simulink model "mrefrobotarm_modified_previous_y_previous_u_previous_ref_pert_2"  (R2018b)
settings: Solver=FixedStepAuto  StartTime=0.0  StopTime=60  RelTol=1e-3  AbsTol=1e-6
undefined symbols (not defined in the file or in its folder): cc, options
libraries: neural x858, simulink x1
(part 12 of 32)

== system mrefrobotarm_modified_previous_y_previous_u_previous_ref_pert_2/m=0 sd=0.001/Layer 3/Delays 1 ==
  "p{3}" : Inport  PortDimensions=30
      mask Display: e = 0.06;c1 = [120 230 180]/255;c2 = ([120 230 180]+0)/(256+128);c3 = ([120 230 180]+128)/(256+128);patch([0 1 1 0],[0 0 1 1],c1);patch([0 1 1 1-e 1-e 0+e],[0 0 1 1-e 0+e 0+e],c2);patch([0 0 1 1-e 0+e 0+e],[0 1 1 1-e 1-e 0+e],c3);plot([0 1 1 0 0],[0 0 1 1 0]);
  mux : Mux  Inputs=1
      mask Display: e = 0.06;c1 = [120 150 230]/255;c2 = ([120 150 230]+0)/383;c3 = ([120 150 230]+128)/383;patch([0 1 1 0],[0 0 1 1],c1);patch([0 1 1 1-e 1-e 0+e],[0 0 1 1-e 0+e 0+e],c2);patch([0 0 1 1-e 0+e 0+e],[0 1 1 1-e 1-e 0+e],c3);plot([0 1 1 0 0],[0 0 1 1 0]);disp('Mux')
  "pd{3,2}" : Outport
      mask Display: e = 0.06;c1 = [120 230 180]/255;c2 = ([120 230 180]+0)/(256+128);c3 = ([120 230 180]+128)/(256+128);patch([0 1 1 0],[0 0 1 1],c1);patch([0 1 1 1-e 1-e 0+e],[0 0 1 1-e 0+e 0+e],c2);patch([0 0 1 1-e 0+e 0+e],[0 1 1 1-e 1-e 0+e],c3);plot([0 1 1 0 0],[0 0 1 1 0]);
  wires:
  "p{3}"/1 -> mux/1
  mux/1 -> "pd{3,2}"/1

== system mrefrobotarm_modified_previous_y_previous_u_previous_ref_pert_2/m=0 sd=0.001/Layer 3/LW{3,2} ==
  "ad{3,2}" : Inport  PortDimensions=30
      mask Display: e = 0.06;c1 = [120 230 180]/255;c2 = ([120 230 180]+0)/(256+128);c3 = ([120 230 180]+128)/(256+128);patch([0 1 1 0],[0 0 1 1],c1);patch([0 1 1 1-e 1-e 0+e],[0 0 1 1-e 0+e 0+e],c2);patch([0 0 1 1-e 0+e 0+e],[0 1 1 1-e 1-e 0+e],c3);plot([0 1 1 0 0],[0 0 1 1 0]);
  "IW{3,2}(1,:)'" : Constant  Value=[-0.1402055465054231897514824822792434133589267730712890625;-0.010591721623553325415389991803749580867588520050048828125;0.66868572840284390412790571645018644630908966064453125;0.06398114714037583805605891029699705541133880615234375;-0.86465249332831961570633438896038569509983062744140625;0.048965740146590712444929494040479767136275768280029296875;0.047539519471818426910036947674598195590078830718994140625;-0.000811648651889989897374733107682232002844102680683135986328125;-0.07220612320831516772745573007341590709984302520751953125;-0.004400076237482670842016130308138599502854049205780029296875;0.1681411013462606185431269523178343661129474639892578125;0.004181807301644306813781515330674665165133774280548095703125;-0.09604306957504916975043585125604295171797275543212890625;0.060371941228756102748587153428161400370299816131591796875;-0.08518750929112839376244892264367081224918365478515625;0.08387689823384537890493817258175113238394260406494140625;0.09173039800025269141503514447322231717407703399658203125;-0.054388580045975111476597163573387661017477512359619140625;0.224529138177710141377474428736604750156402587890625;0.0421708309152450666612566010371665470302104949951171875;-0.051414827892769028594432967338434536941349506378173828125;0.62790175807750536751683512193267233669757843017578125;-0.2698100128415774623391598652233369648456573486328125;-0.396414898341079957599930594369652681052684783935546875;0.09967094816048416294762546385754831135272979736328125;-0.100367342611018928177912812316208146512508392333984375;0.00366898647383644138653124855409259907901287078857421875;0.1491506044864047975107013144224765710532665252685546875;0.0841762454661753312112892899676808156073093414306640625;0.0259526344866221024554331364697645767591893672943115234375]
      mask Display: e = 0.06;c1 = [120 150 230]/255;c2 = ([120 150 230]+0)/383;c3 = ([120 150 230]+128)/383;patch([0 1 1 0],[0 0 1 1],c1);patch([0 1 1 1-e 1-e 0+e],[0 0 1 1-e 0+e 0+e],c2);patch([0 0 1 1-e 0+e 0+e],[0 1 1 1-e 1-e 0+e],c3);plot([0 1 1 0 0],[0 0 1 1 0]);disp('weights');
  Mux : Mux  Inputs=1
      mask Display: e = 0.06;c1 = [120 150 230]/255;c2 = ([120 150 230]+0)/383;c3 = ([120 150 230]+128)/383;patch([0 1 1 0],[0 0 1 1],c1);patch([0 1 1 1-e 1-e 0+e],[0 0 1 1-e 0+e 0+e],c2);patch([0 0 1 1-e 0+e 0+e],[0 1 1 1-e 1-e 0+e],c3);plot([0 1 1 0 0],[0 0 1 1 0]);disp('Mux');
  dotprod1 : neural/Weight Functions/dotprod
  "lz{3,2}" : Outport
      mask Display: e = 0.06;c1 = [120 230 180]/255;c2 = ([120 230 180]+0)/(256+128);c3 = ([120 230 180]+128)/(256+128);patch([0 1 1 0],[0 0 1 1],c1);patch([0 1 1 1-e 1-e 0+e],[0 0 1 1-e 0+e 0+e],c2);patch([0 0 1 1-e 0+e 0+e],[0 1 1 1-e 1-e 0+e],c3);plot([0 1 1 0 0],[0 0 1 1 0]);
  wires:
  "IW{3,2}(1,:)'"/1 -> dotprod1/1
  "ad{3,2}"/1 -> dotprod1/2
  dotprod1/1 -> Mux/1
  Mux/1 -> "lz{3,2}"/1

== system mrefrobotarm_modified_previous_y_previous_u_previous_ref_pert_2/m=0 sd=0.01/Layer 1/Delays 1 ==
  "p{1}" : Inport  PortDimensions=10
      mask Display: e = 0.06;c1 = [120 230 180]/255;c2 = ([120 230 180]+0)/(256+128);c3 = ([120 230 180]+128)/(256+128);patch([0 1 1 0],[0 0 1 1],c1);patch([0 1 1 1-e 1-e 0+e],[0 0 1 1-e 0+e 0+e],c2);patch([0 0 1 1-e 0+e 0+e],[0 1 1 1-e 1-e 0+e],c3);plot([0 1 1 0 0],[0 0 1 1 0]);
  mux : Mux  Inputs=1
      mask Display: e = 0.06;c1 = [120 150 230]/255;c2 = ([120 150 230]+0)/383;c3 = ([120 150 230]+128)/383;patch([0 1 1 0],[0 0 1 1],c1);patch([0 1 1 1-e 1-e 0+e],[0 0 1 1-e 0+e 0+e],c2);patch([0 0 1 1-e 0+e 0+e],[0 1 1 1-e 1-e 0+e],c3);plot([0 1 1 0 0],[0 0 1 1 0]);disp('Mux')
  "pd{1,1}" : Outport
      mask Display: e = 0.06;c1 = [120 230 180]/255;c2 = ([120 230 180]+0)/(256+128);c3 = ([120 230 180]+128)/(256+128);patch([0 1 1 0],[0 0 1 1],c1);patch([0 1 1 1-e 1-e 0+e],[0 0 1 1-e 0+e 0+e],c2);patch([0 0 1 1-e 0+e 0+e],[0 1 1 1-e 1-e 0+e],c3);plot([0 1 1 0 0],[0 0 1 1 0]);
  wires:
  "p{1}"/1 -> mux/1
  mux/1 -> "pd{1,1}"/1

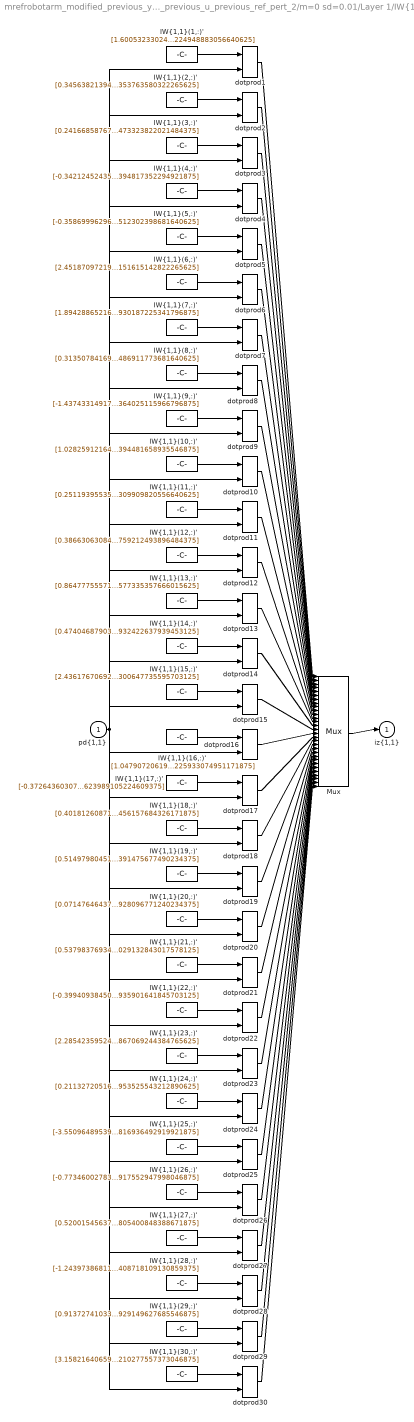
== system mrefrobotarm_modified_previous_y_previous_u_previous_ref_pert_2/m=0 sd=0.01/Layer 1/IW{1,1} ==
  "pd{1,1}" : Inport  PortDimensions=10
      mask Display: e = 0.06;c1 = [120 230 180]/255;c2 = ([120 230 180]+0)/(256+128);c3 = ([120 230 180]+128)/(256+128);patch([0 1 1 0],[0 0 1 1],c1);patch([0 1 1 1-e 1-e 0+e],[0 0 1 1-e 0+e 0+e],c2);patch([0 0 1 1-e 0+e 0+e],[0 1 1 1-e 1-e 0+e],c3);plot([0 1 1 0 0],[0 0 1 1 0]);
  "IW{1,1}(1,:)'" : Constant  Value=[1.6005323302449576683414989020093344151973724365234375;-0.417552450811128128549398752511478960514068603515625;0.55193056340048218810778735132771544158458709716796875;-1.656844648544015807800633410806767642498016357421875;-0.445156872313967111320920366779319010674953460693359375;-0.357993656785643488138504153539543040096759796142578125;0.8075036988304555851669874755316413938999176025390625;0.32933748752871350173876408007345162332057952880859375;-1.098390333069939828192218556068837642669677734375;0.59384595790079830468499721973785199224948883056640625]
      mask Display: e = 0.06;c1 = [120 150 230]/255;c2 = ([120 150 230]+0)/383;c3 = ([120 150 230]+128)/383;patch([0 1 1 0],[0 0 1 1],c1);patch([0 1 1 1-e 1-e 0+e],[0 0 1 1-e 0+e 0+e],c2);patch([0 0 1 1-e 0+e 0+e],[0 1 1 1-e 1-e 0+e],c3);plot([0 1 1 0 0],[0 0 1 1 0]);disp('Weights');
  "IW{1,1}(10,:)'" : Constant  Value=[1.0282591216485474916453313198871910572052001953125;-0.9394700415261623138718505288125015795230865478515625;-0.1464072774747041394416413595536141656339168548583984375;0.35893683894597583350360991971683688461780548095703125;0.63803398415225121009797248916584067046642303466796875;-0.6584107764562883158276918038609437644481658935546875;0.224345789764162584223328167354338802397251129150390625;-0.104869593344576739202267390282941050827503204345703125;0.058368077947360895441075712142264819703996181488037109375;-0.476899899624756595795105340584996156394481658935546875]
      mask Display: e = 0.06;c1 = [120 150 230]/255;c2 = ([120 150 230]+0)/383;c3 = ([120 150 230]+128)/383;patch([0 1 1 0],[0 0 1 1],c1);patch([0 1 1 1-e 1-e 0+e],[0 0 1 1-e 0+e 0+e],c2);patch([0 0 1 1-e 0+e 0+e],[0 1 1 1-e 1-e 0+e],c3);plot([0 1 1 0 0],[0 0 1 1 0]);disp('Weights');
  "IW{1,1}(11,:)'" : Constant  Value=[0.2511939553542792413765027959016151726245880126953125;0.0304852076696646955011882340613738051615655422210693359375;0.08979694144875320638288229702084208838641643524169921875;1.45524334878463701414830211433582007884979248046875;0.257452735606438387616634599908138625323772430419921875;0.69756328904774778099096010919311083853244781494140625;1.2591851632830575180577170613105408847332000732421875;-1.1843458045774484244105906327604316174983978271484375;-0.308791981279867455700838263510377146303653717041015625;-0.1644213236704926972553408859312185086309909820556640625]
      mask Display: e = 0.06;c1 = [120 150 230]/255;c2 = ([120 150 230]+0)/383;c3 = ([120 150 230]+128)/383;patch([0 1 1 0],[0 0 1 1],c1);patch([0 1 1 1-e 1-e 0+e],[0 0 1 1-e 0+e 0+e],c2);patch([0 0 1 1-e 0+e 0+e],[0 1 1 1-e 1-e 0+e],c3);plot([0 1 1 0 0],[0 0 1 1 0]);disp('Weights');
  "IW{1,1}(12,:)'" : Constant  Value=[0.38663063084623716658683179048239253461360931396484375;0.281806448988240976216701483281212858855724334716796875;0.5896989095744089581785374321043491363525390625;0.06562069683940370545816023195584421046078205108642578125;-0.50622558401284578621925902552902698516845703125;0.182093229094074604557107477376121096312999725341796875;-0.6983018957877054067040489826467819511890411376953125;0.438583607355719495846102518044062890112400054931640625;1.322440379673329058363151489174924790859222412109375;0.9185640257197904556818457422195933759212493896484375]
      mask Display: e = 0.06;c1 = [120 150 230]/255;c2 = ([120 150 230]+0)/383;c3 = ([120 150 230]+128)/383;patch([0 1 1 0],[0 0 1 1],c1);patch([0 1 1 1-e 1-e 0+e],[0 0 1 1-e 0+e 0+e],c2);patch([0 0 1 1-e 0+e 0+e],[0 1 1 1-e 1-e 0+e],c3);plot([0 1 1 0 0],[0 0 1 1 0]);disp('Weights');
  "IW{1,1}(13,:)'" : Constant  Value=[0.8647775557185017891725919980672188103199005126953125;0.7011154199989448887464504878153093159198760986328125;-0.400894445693125878182883070621755905449390411376953125;-0.85589349137761361330234421984641812741756439208984375;-1.222171594976523056885753248934634029865264892578125;-1.0803728679097612808135409068199805915355682373046875;1.152315806126472441661690027103759348392486572265625;-0.60725041429012549532018283571233041584491729736328125;0.465618029094280683199968962071579881012439727783203125;-0.700323189074508523077611243934370577335357666015625]
      mask Display: e = 0.06;c1 = [120 150 230]/255;c2 = ([120 150 230]+0)/383;c3 = ([120 150 230]+128)/383;patch([0 1 1 0],[0 0 1 1],c1);patch([0 1 1 1-e 1-e 0+e],[0 0 1 1-e 0+e 0+e],c2);patch([0 0 1 1-e 0+e 0+e],[0 1 1 1-e 1-e 0+e],c3);plot([0 1 1 0 0],[0 0 1 1 0]);disp('Weights');
  "IW{1,1}(14,:)'" : Constant  Value=[0.47404687903363373902010380334104411303997039794921875;-0.24339277626495003925555238311062566936016082763671875;0.041616970055157687102820318614249117672443389892578125;-0.67343257839028136668702018141630105674266815185546875;-0.22538734328270881857037011286593042314052581787109375;-0.6426922803930679162220940270344726741313934326171875;0.83286259191018985337251478995312936604022979736328125;0.33559175668810470316572036608704365789890289306640625;-0.0999840650353143178818982050870545208454132080078125;0.01297536616560969642553136083051867899484932422637939453125]
      mask Display: e = 0.06;c1 = [120 150 230]/255;c2 = ([120 150 230]+0)/383;c3 = ([120 150 230]+128)/383;patch([0 1 1 0],[0 0 1 1],c1);patch([0 1 1 1-e 1-e 0+e],[0 0 1 1-e 0+e 0+e],c2);patch([0 0 1 1-e 0+e 0+e],[0 1 1 1-e 1-e 0+e],c3);plot([0 1 1 0 0],[0 0 1 1 0]);disp('Weights');
  "IW{1,1}(15,:)'" : Constant  Value=[2.436176706929539026447173455380834639072418212890625;-2.4094755348923566629082415602169930934906005859375;-0.005007248187668153320550867846350229228846728801727294921875;-0.47412315155033357694236428869771771132946014404296875;-0.239072874588061645706460467408760450780391693115234375;-0.48929756932282064685324485253659076988697052001953125;0.34953248476371145958552233423688448965549468994140625;0.08441204920994031801750878685197676531970500946044921875;0.1438827592365415075637002928488072939217090606689453125;-0.004157588195574994822945047445728050661273300647735595703125]
      mask Display: e = 0.06;c1 = [120 150 230]/255;c2 = ([120 150 230]+0)/383;c3 = ([120 150 230]+128)/383;patch([0 1 1 0],[0 0 1 1],c1);patch([0 1 1 1-e 1-e 0+e],[0 0 1 1-e 0+e 0+e],c2);patch([0 0 1 1-e 0+e 0+e],[0 1 1 1-e 1-e 0+e],c3);plot([0 1 1 0 0],[0 0 1 1 0]);disp('Weights');
  "IW{1,1}(16,:)'" : Constant  Value=[1.0479072061917804603581316769123077392578125;-1.188325342910974580235006214934401214122772216796875;0.08282680037954197327376704151902231387794017791748046875;-0.0750577313756301822689209757299977354705333709716796875;-0.5892561557388578119542899003135971724987030029296875;0.71866424561459663067353176302276551723480224609375;-0.22523367428440110860066170062054879963397979736328125;0.020095498778328953204397322451768559403717517852783203125;0.6224434774035072504005938753834925591945648193359375;0.78975562256306985897680306152324192225933074951171875]
      mask Display: e = 0.06;c1 = [120 150 230]/255;c2 = ([120 150 230]+0)/383;c3 = ([120 150 230]+128)/383;patch([0 1 1 0],[0 0 1 1],c1);patch([0 1 1 1-e 1-e 0+e],[0 0 1 1-e 0+e 0+e],c2);patch([0 0 1 1-e 0+e 0+e],[0 1 1 1-e 1-e 0+e],c3);plot([0 1 1 0 0],[0 0 1 1 0]);disp('Weights');
  "IW{1,1}(17,:)'" : Constant  Value=[-0.3726436030766275830927725110086612403392791748046875;0.11258683397342060528156792997833690606057643890380859375;-0.289959409428568459787811661954037845134735107421875;-1.031936087352059328026143703027628362178802490234375;-0.1005469337870905921494824042383697815239429473876953125;-0.7886302451998832285795515417703427374362945556640625;-1.2097660984615414836440550061524845659732818603515625;1.3304332530030347214733410510234534740447998046875;-0.358596909644648409454248394467867910861968994140625;-0.7905800103699822667380203711218200623989105224609375]
      mask Display: e = 0.06;c1 = [120 150 230]/255;c2 = ([120 150 230]+0)/383;c3 = ([120 150 230]+128)/383;patch([0 1 1 0],[0 0 1 1],c1);patch([0 1 1 1-e 1-e 0+e],[0 0 1 1-e 0+e 0+e],c2);patch([0 0 1 1-e 0+e 0+e],[0 1 1 1-e 1-e 0+e],c3);plot([0 1 1 0 0],[0 0 1 1 0]);disp('Weights');
  "IW{1,1}(18,:)'" : Constant  Value=[0.40181260871088830821662440939689986407756805419921875;-0.3655278381722830705058413514052517712116241455078125;-0.3887665115315057651201868793577887117862701416015625;0.1255625700217244677947547870644484646618366241455078125;1.3364495829600182563723365092300809919834136962890625;-0.52340776552323420300893985768198035657405853271484375;-1.31475125145500815193599919439293444156646728515625;-1.3538114546953365913140032716910354793071746826171875;1.38302121689699664131012468715198338031768798828125;1.6711842678573827214449920575134456157684326171875]
      mask Display: e = 0.06;c1 = [120 150 230]/255;c2 = ([120 150 230]+0)/383;c3 = ([120 150 230]+128)/383;patch([0 1 1 0],[0 0 1 1],c1);patch([0 1 1 1-e 1-e 0+e],[0 0 1 1-e 0+e 0+e],c2);patch([0 0 1 1-e 0+e 0+e],[0 1 1 1-e 1-e 0+e],c3);plot([0 1 1 0 0],[0 0 1 1 0]);disp('Weights');
  "IW{1,1}(19,:)'" : Constant  Value=[0.51497980451554870029440280632115900516510009765625;-1.42085629222442921815172667265869677066802978515625;1.0391866609251596553775698339450173079967498779296875;1.106976984444728362433352231164462864398956298828125;-0.35113070885377950514083522648434154689311981201171875;-0.7069018467434926566994590757531113922595977783203125;-0.254139746779877329085906012551276944577693939208984375;-0.7248155119095540666052102096728049218654632568359375;0.374266881528209582885580175570794381201267242431640625;0.330929099275292182280594488474889658391475677490234375]
      mask Display: e = 0.06;c1 = [120 150 230]/255;c2 = ([120 150 230]+0)/383;c3 = ([120 150 230]+128)/383;patch([0 1 1 0],[0 0 1 1],c1);patch([0 1 1 1-e 1-e 0+e],[0 0 1 1-e 0+e 0+e],c2);patch([0 0 1 1-e 0+e 0+e],[0 1 1 1-e 1-e 0+e],c3);plot([0 1 1 0 0],[0 0 1 1 0]);disp('Weights');
  "IW{1,1}(2,:)'" : Constant  Value=[0.345638213943738337174949037944315932691097259521484375;0.195583616221133793633413233692408539354801177978515625;0.1344595428584056950871428171012667007744312286376953125;-1.23287629498543527262199859251268208026885986328125;-0.83660373021310174834752615424804389476776123046875;-0.88071706507825098242392414249479770660400390625;-0.50793809907330034203454260932630859315395355224609375;-0.3209031093734238115899870535940863192081451416015625;-0.99619019638493877533136355850729160010814666748046875;-0.1224679396658378272011447052136645652353763580322265625]
      mask Display: e = 0.06;c1 = [120 150 230]/255;c2 = ([120 150 230]+0)/383;c3 = ([120 150 230]+128)/383;patch([0 1 1 0],[0 0 1 1],c1);patch([0 1 1 1-e 1-e 0+e],[0 0 1 1-e 0+e 0+e],c2);patch([0 0 1 1-e 0+e 0+e],[0 1 1 1-e 1-e 0+e],c3);plot([0 1 1 0 0],[0 0 1 1 0]);disp('Weights');
  "IW{1,1}(20,:)'" : Constant  Value=[0.071476464372509040945402603028924204409122467041015625;-1.3396188282270775626869863117462955415248870849609375;-0.47342514154079362587168589016073383390903472900390625;0.416476577299325523284778682864271104335784912109375;0.554704532946700634710168742458336055278778076171875;-0.07716201523714248666774295770665048621594905853271484375;-0.6155064445532258954330018241307698190212249755859375;-0.51446038660242654483312207958078943192958831787109375;2.007930354311708409653647322556935250759124755859375;0.34230669970004734548041369635029695928096771240234375]
      mask Display: e = 0.06;c1 = [120 150 230]/255;c2 = ([120 150 230]+0)/383;c3 = ([120 150 230]+128)/383;patch([0 1 1 0],[0 0 1 1],c1);patch([0 1 1 1-e 1-e 0+e],[0 0 1 1-e 0+e 0+e],c2);patch([0 0 1 1-e 0+e 0+e],[0 1 1 1-e 1-e 0+e],c3);plot([0 1 1 0 0],[0 0 1 1 0]);disp('Weights');
  "IW{1,1}(21,:)'" : Constant  Value=[0.5379837693477023119470459278090856969356536865234375;-0.05957890286965293602516879900576896034181118011474609375;-0.18289215056864327468844066970632411539554595947265625;-0.5118414567849498553187004290521144866943359375;-0.8059454900675933064491118784644640982151031494140625;-0.11815798259500599753923921753084869123995304107666015625;0.68352163379281716260038592736236751079559326171875;0.2144653787375029596606879067621775902807712554931640625;0.008114355246120578957214064530489849857985973358154296875;0.04031370499444593413773674228650634177029132843017578125]
      mask Display: e = 0.06;c1 = [120 150 230]/255;c2 = ([120 150 230]+0)/383;c3 = ([120 150 230]+128)/383;patch([0 1 1 0],[0 0 1 1],c1);patch([0 1 1 1-e 1-e 0+e],[0 0 1 1-e 0+e 0+e],c2);patch([0 0 1 1-e 0+e 0+e],[0 1 1 1-e 1-e 0+e],c3);plot([0 1 1 0 0],[0 0 1 1 0]);disp('Weights');
  "IW{1,1}(22,:)'" : Constant  Value=[-0.399409384502136532990590467306901700794696807861328125;0.10413271486194959625226630350880441255867481231689453125;0.545146184915891840461199535639025270938873291015625;0.340093448222392902291488780974759720265865325927734375;-0.47095834251783674773150778491981327533721923828125;1.29070041007550617706556295161135494709014892578125;-0.67087188612048087588135558689828030765056610107421875;-0.04682306432685011399197350101530901156365871429443359375;0.5567769195740022158958026921027339994907379150390625;0.80826068824523755740329988839221186935901641845703125]
      mask Display: e = 0.06;c1 = [120 150 230]/255;c2 = ([120 150 230]+0)/383;c3 = ([120 150 230]+128)/383;patch([0 1 1 0],[0 0 1 1],c1);patch([0 1 1 1-e 1-e 0+e],[0 0 1 1-e 0+e 0+e],c2);patch([0 0 1 1-e 0+e 0+e],[0 1 1 1-e 1-e 0+e],c3);plot([0 1 1 0 0],[0 0 1 1 0]);disp('Weights');
  "IW{1,1}(23,:)'" : Constant  Value=[2.285423595247963124421630709548480808734893798828125;-0.67606217603436091767576954225660301744937896728515625;-1.033615614828911066780392502550967037677764892578125;0.5232288854111846188033041471499018371105194091796875;0.38509848841146443465532911432092078030109405517578125;-0.256968841229491429256626133792451582849025726318359375;0.415105426631309837315342292640707455575466156005859375;0.5870312160049702132624815931194461882114410400390625;-1.74917018356650100230353928054682910442352294921875;-0.58845798863241915999111597557202912867069244384765625]
      mask Display: e = 0.06;c1 = [120 150 230]/255;c2 = ([120 150 230]+0)/383;c3 = ([120 150 230]+128)/383;patch([0 1 1 0],[0 0 1 1],c1);patch([0 1 1 1-e 1-e 0+e],[0 0 1 1-e 0+e 0+e],c2);patch([0 0 1 1-e 0+e 0+e],[0 1 1 1-e 1-e 0+e],c3);plot([0 1 1 0 0],[0 0 1 1 0]);disp('Weights');
  "IW{1,1}(24,:)'" : Constant  Value=[0.2113272051696663822450972247679601423442363739013671875;0.8700963983258105383100655672024004161357879638671875;0.10133326278470915216001202452389406971633434295654296875;-0.82496897474394736970992880742414854466915130615234375;-0.3134736277608300980546118807978928089141845703125;-0.328835142809582758882669395461562089622020721435546875;-0.3023265515330761932233372135669924318790435791015625;-0.16758057479458809968519972244394011795520782470703125;-1.0185128834635255312690560458577238023281097412109375;-0.21937198871722396464889470735215581953525543212890625]
      mask Display: e = 0.06;c1 = [120 150 230]/255;c2 = ([120 150 230]+0)/383;c3 = ([120 150 230]+128)/383;patch([0 1 1 0],[0 0 1 1],c1);patch([0 1 1 1-e 1-e 0+e],[0 0 1 1-e 0+e 0+e],c2);patch([0 0 1 1-e 0+e 0+e],[0 1 1 1-e 1-e 0+e],c3);plot([0 1 1 0 0],[0 0 1 1 0]);disp('Weights');
  "IW{1,1}(25,:)'" : Constant  Value=[-3.550964895399927545582841048599220812320709228515625;2.241874250461567186221145675517618656158447265625;0.132149124365854631069083779948414303362369537353515625;-0.2422445058906708970081211873548454605042934417724609375;0.89656360913103505527743664060835726559162139892578125;-0.353976488302861103107943563372828066349029541015625;0.720322560666469602352890433394350111484527587890625;0.36801503579594452286727346290717832744121551513671875;-0.0803012567947585520489184318648767657577991485595703125;-0.2356022687239746893350655909671331755816936492919921875]
      mask Display: e = 0.06;c1 = [120 150 230]/255;c2 = ([120 150 230]+0)/383;c3 = ([120 150 230]+128)/383;patch([0 1 1 0],[0 0 1 1],c1);patch([0 1 1 1-e 1-e 0+e],[0 0 1 1-e 0+e 0+e],c2);patch([0 0 1 1-e 0+e 0+e],[0 1 1 1-e 1-e 0+e],c3);plot([0 1 1 0 0],[0 0 1 1 0]);disp('Weights');
  "IW{1,1}(26,:)'" : Constant  Value=[-0.77346002783295231264304447904578410089015960693359375;0.210490320262209540391751261267927475273609161376953125;0.1595722891588296776799182907780050300061702728271484375;0.44625282393541432224282061724807135760784149169921875;0.93453436903255171497306719174957834184169769287109375;-0.274651577897329357558220408463967032730579376220703125;-0.5927690250574275676598290374386124312877655029296875;-0.03486262132694850635061811772175133228302001953125;1.8315525895444870752015731341089121997356414794921875;0.56898405222457337782060449171694926917552947998046875]
      mask Display: e = 0.06;c1 = [120 150 230]/255;c2 = ([120 150 230]+0)/383;c3 = ([120 150 230]+128)/383;patch([0 1 1 0],[0 0 1 1],c1);patch([0 1 1 1-e 1-e 0+e],[0 0 1 1-e 0+e 0+e],c2);patch([0 0 1 1-e 0+e 0+e],[0 1 1 1-e 1-e 0+e],c3);plot([0 1 1 0 0],[0 0 1 1 0]);disp('Weights');
  "IW{1,1}(27,:)'" : Constant  Value=[0.52001545637661961141162692001671530306339263916015625;-1.136503515664809782492739032022655010223388671875;-0.012356381719821916964630048596518463455140590667724609375;0.32379264286014375340272408720920793712139129638671875;-0.424148125090513306023609629846760071814060211181640625;-0.80277728372693391012404617868014611303806304931640625;-0.698777100324295741273772364365868270397186279296875;-0.92985628839251777133512177897500805556774139404296875;1.125322950545620148687930850428529083728790283203125;-0.278550256307673549382997180146048776805400848388671875]
      mask Display: e = 0.06;c1 = [120 150 230]/255;c2 = ([120 150 230]+0)/383;c3 = ([120 150 230]+128)/383;patch([0 1 1 0],[0 0 1 1],c1);patch([0 1 1 1-e 1-e 0+e],[0 0 1 1-e 0+e 0+e],c2);patch([0 0 1 1-e 0+e 0+e],[0 1 1 1-e 1-e 0+e],c3);plot([0 1 1 0 0],[0 0 1 1 0]);disp('Weights');
  "IW{1,1}(28,:)'" : Constant  Value=[-1.243973868112619118875272761215455830097198486328125;1.4053848550015508589439150455291382968425750732421875;0.356800221457132138436207924314658157527446746826171875;-0.149489257045333945317366897143074311316013336181640625;0.396534450900142443341422904268256388604640960693359375;-0.77587114554228764351506697494187392294406890869140625;0.61822090940689300442301146176760084927082061767578125;0.413520766322310551199592509874491952359676361083984375;0.021180723707641076203334051797355641610920429229736328125;-0.9403622899705579296636415165266953408718109130859375]
      mask Display: e = 0.06;c1 = [120 150 230]/255;c2 = ([120 150 230]+0)/383;c3 = ([120 150 230]+128)/383;patch([0 1 1 0],[0 0 1 1],c1);patch([0 1 1 1-e 1-e 0+e],[0 0 1 1-e 0+e 0+e],c2);patch([0 0 1 1-e 0+e 0+e],[0 1 1 1-e 1-e 0+e],c3);plot([0 1 1 0 0],[0 0 1 1 0]);disp('Weights');
  "IW{1,1}(29,:)'" : Constant  Value=[0.9137274103399610769571381752029992640018463134765625;-0.4448377030389110142749586884747259318828582763671875;0.0392184877779516438689455526400706730782985687255859375;0.35633029255421166947570554839330725371837615966796875;-0.688939789786528589132785782567225396633148193359375;-0.323380977820002690759082497606868855655193328857421875;0.86933585346985620123660964964074082672595977783203125;-0.6538605389731426686950044313562102615833282470703125;-1.4304009218130619984776785713620483875274658203125;-1.065350411555140208719194561126641929149627685546875]
      mask Display: e = 0.06;c1 = [120 150 230]/255;c2 = ([120 150 230]+0)/383;c3 = ([120 150 230]+128)/383;patch([0 1 1 0],[0 0 1 1],c1);patch([0 1 1 1-e 1-e 0+e],[0 0 1 1-e 0+e 0+e],c2);patch([0 0 1 1-e 0+e 0+e],[0 1 1 1-e 1-e 0+e],c3);plot([0 1 1 0 0],[0 0 1 1 0]);disp('Weights');
  "IW{1,1}(3,:)'" : Constant  Value=[0.2416685876718483172442830664294888265430927276611328125;0.0252694618995373543324234333340427838265895843505859375;-0.41844675079042037424414957058615982532501220703125;0.75703934561817065596045495112775824964046478271484375;-0.703839563216872132755952407023869454860687255859375;-0.099282164737776013030412514126510359346866607666015625;0.0888071779512836501080386142348288558423519134521484375;-0.50997529536766961211213811111520044505596160888671875;0.60609555056473685130669082354870624840259552001953125;0.6622528225229602494295022552250884473323822021484375]
      mask Display: e = 0.06;c1 = [120 150 230]/255;c2 = ([120 150 230]+0)/383;c3 = ([120 150 230]+128)/383;patch([0 1 1 0],[0 0 1 1],c1);patch([0 1 1 1-e 1-e 0+e],[0 0 1 1-e 0+e 0+e],c2);patch([0 0 1 1-e 0+e 0+e],[0 1 1 1-e 1-e 0+e],c3);plot([0 1 1 0 0],[0 0 1 1 0]);disp('Weights');
  "IW{1,1}(30,:)'" : Constant  Value=[3.158216406599627656959228261257521808147430419921875;-3.64954501760108751540201410534791648387908935546875;0.06286162761835974166491070036499877460300922393798828125;0.89385880454740795908463724117609672248363494873046875;0.8846381083262235822672892027185298502445220947265625;-0.8855804214017546360793176063452847301959991455078125;0.4204648159002488672086883525480516254901885986328125;-0.251539163660401021704871027395711280405521392822265625;0.293698855570228734013227267496404238045215606689453125;-0.9864148010077424810759794127079658210277557373046875]
      mask Display: e = 0.06;c1 = [120 150 230]/255;c2 = ([120 150 230]+0)/383;c3 = ([120 150 230]+128)/383;patch([0 1 1 0],[0 0 1 1],c1);patch([0 1 1 1-e 1-e 0+e],[0 0 1 1-e 0+e 0+e],c2);patch([0 0 1 1-e 0+e 0+e],[0 1 1 1-e 1-e 0+e],c3);plot([0 1 1 0 0],[0 0 1 1 0]);disp('Weights');
  "IW{1,1}(4,:)'" : Constant  Value=[-0.342124524350444880749222420490696094930171966552734375;-0.331637133412337081761478430053102783858776092529296875;-0.253587678375058356294857730972580611705780029296875;1.61278015133414331927497187280096113681793212890625;0.634229067833477433424604896572418510913848876953125;1.6408195518074843999301037911209277808666229248046875;-0.1641419536002190204815320839770720340311527252197265625;0.8100441301801011295680154944420792162418365478515625;-0.50509883718888948234138069892651401460170745849609375;0.69791960577225331530115681744064204394817352294921875]
      mask Display: e = 0.06;c1 = [120 150 230]/255;c2 = ([120 150 230]+0)/383;c3 = ([120 150 230]+128)/383;patch([0 1 1 0],[0 0 1 1],c1);patch([0 1 1 1-e 1-e 0+e],[0 0 1 1-e 0+e 0+e],c2);patch([0 0 1 1-e 0+e 0+e],[0 1 1 1-e 1-e 0+e],c3);plot([0 1 1 0 0],[0 0 1 1 0]);disp('Weights');
  "IW{1,1}(5,:)'" : Constant  Value=[-0.35869996296015305148330298834480345249176025390625;1.7021189283291200400327625175123102962970733642578125;-0.56932964436483579628855977716739289462566375732421875;0.71737968417619712990784819339751265943050384521484375;0.68459003758094028047054280250449664890766143798828125;1.2303897595502417683377416324219666421413421630859375;-0.784478655065325991557756424299441277980804443359375;0.66041658341854747593657748438999988138675689697265625;0.50436912549123225080194288238999433815479278564453125;1.2823390693166063503127816147753037512302398681640625]
      mask Display: e = 0.06;c1 = [120 150 230]/255;c2 = ([120 150 230]+0)/383;c3 = ([120 150 230]+128)/383;patch([0 1 1 0],[0 0 1 1],c1);patch([0 1 1 1-e 1-e 0+e],[0 0 1 1-e 0+e 0+e],c2);patch([0 0 1 1-e 0+e 0+e],[0 1 1 1-e 1-e 0+e],c3);plot([0 1 1 0 0],[0 0 1 1 0]);disp('Weights');
  "IW{1,1}(6,:)'" : Constant  Value=[2.45187097219104810363887736457400023937225341796875;-1.8475031130362389308885440186713822185993194580078125;-0.977866748710544353428986141807399690151214599609375;-0.186041305079257923704716404245118610560894012451171875;-0.8003281333951626219658237459952943027019500732421875;0.55623890223238114938197895753546617925167083740234375;-0.30295428428282245025826568962656892836093902587890625;0.4205587896920566226555138200637884438037872314453125;-0.56915030951236733613995966152288019657135009765625;0.676291589005535431766702458844520151615142822265625]
      mask Display: e = 0.06;c1 = [120 150 230]/255;c2 = ([120 150 230]+0)/383;c3 = ([120 150 230]+128)/383;patch([0 1 1 0],[0 0 1 1],c1);patch([0 1 1 1-e 1-e 0+e],[0 0 1 1-e 0+e 0+e],c2);patch([0 0 1 1-e 0+e 0+e],[0 1 1 1-e 1-e 0+e],c3);plot([0 1 1 0 0],[0 0 1 1 0]);disp('Weights');
  "IW{1,1}(7,:)'" : Constant  Value=[1.8942886521650648123937799027771688997745513916015625;-0.201095404734635108123796953805140219628810882568359375;-1.2176469214736649337993412700598128139972686767578125;0.0107793928178477223245312899280179408378899097442626953125;1.008179727227366928588025984936393797397613525390625;-1.26206897378698812417496810667216777801513671875;-0.008277865165198981800553923449115245603024959564208984375;-0.458622399203354180752256752384710125625133514404296875;-0.0270560261847352656605636411768500693142414093017578125;0.462354666451655293979428051898139528930187225341796875]
      mask Display: e = 0.06;c1 = [120 150 230]/255;c2 = ([120 150 230]+0)/383;c3 = ([120 150 230]+128)/383;patch([0 1 1 0],[0 0 1 1],c1);patch([0 1 1 1-e 1-e 0+e],[0 0 1 1-e 0+e 0+e],c2);patch([0 0 1 1-e 0+e 0+e],[0 1 1 1-e 1-e 0+e],c3);plot([0 1 1 0 0],[0 0 1 1 0]);disp('Weights');
  "IW{1,1}(8,:)'" : Constant  Value=[0.313507841697646283396494482076377607882022857666015625;1.230369431226223664310737149207852780818939208984375;-0.5693225367655225799268237096839584410190582275390625;0.12425839684622318193074619330218411050736904144287109375;-0.66146302735856188359520047015394084155559539794921875;1.13549454078476497187466520699672400951385498046875;0.79073832094897855693460542170214466750621795654296875;-0.55317000478638511662410337521578185260295867919921875;0.320343258377163209171811786291073076426982879638671875;0.2034404993085831281351971711046644486486911773681640625]
      mask Display: e = 0.06;c1 = [120 150 230]/255;c2 = ([120 150 230]+0)/383;c3 = ([120 150 230]+128)/383;patch([0 1 1 0],[0 0 1 1],c1);patch([0 1 1 1-e 1-e 0+e],[0 0 1 1-e 0+e 0+e],c2);patch([0 0 1 1-e 0+e 0+e],[0 1 1 1-e 1-e 0+e],c3);plot([0 1 1 0 0],[0 0 1 1 0]);disp('Weights');
  "IW{1,1}(9,:)'" : Constant  Value=[-1.437433149170439516950636971159838140010833740234375;1.027625073214063267101892051869072020053863525390625;0.358104370883538525305311850388534367084503173828125;-0.06776579622492635845976138853075099177658557891845703125;0.43654082100812707789572186811710707843303680419921875;0.273980932045105152194963693546014837920665740966796875;-0.6865407783403731922788892916287295520305633544921875;0.0079642785320317467656625609606635407544672489166259765625;1.94403315795498965456999940215609967708587646484375;1.0665439273264343267300091611105017364025115966796875]
      mask Display: e = 0.06;c1 = [120 150 230]/255;c2 = ([120 150 230]+0)/383;c3 = ([120 150 230]+128)/383;patch([0 1 1 0],[0 0 1 1],c1);patch([0 1 1 1-e 1-e 0+e],[0 0 1 1-e 0+e 0+e],c2);patch([0 0 1 1-e 0+e 0+e],[0 1 1 1-e 1-e 0+e],c3);plot([0 1 1 0 0],[0 0 1 1 0]);disp('Weights');
  Mux : Mux  Inputs=30
      mask Display: e = 0.06;c1 = [120 150 230]/255;c2 = ([120 150 230]+0)/383;c3 = ([120 150 230]+128)/383;patch([0 1 1 0],[0 0 1 1],c1);patch([0 1 1 1-e 1-e 0+e],[0 0 1 1-e 0+e 0+e],c2);patch([0 0 1 1-e 0+e 0+e],[0 1 1 1-e 1-e 0+e],c3);plot([0 1 1 0 0],[0 0 1 1 0]);disp('Mux');
  dotprod{1..30} (30 alike) : neural/Weight Functions/dotprod
  "iz{1,1}" : Outport
      mask Display: e = 0.06;c1 = [120 230 180]/255;c2 = ([120 230 180]+0)/(256+128);c3 = ([120 230 180]+128)/(256+128);patch([0 1 1 0],[0 0 1 1],c1);patch([0 1 1 1-e 1-e 0+e],[0 0 1 1-e 0+e 0+e],c2);patch([0 0 1 1-e 0+e 0+e],[0 1 1 1-e 1-e 0+e],c3);plot([0 1 1 0 0],[0 0 1 1 0]);
  wires:
  "IW{1,1}(1,:)'"/1 -> dotprod1/1
  "pd{1,1}"/1 -> dotprod1/2, dotprod2/2, dotprod3/2, dotprod4/2, dotprod5/2, dotprod6/2, dotprod7/2, dotprod8/2, dotprod9/2, dotprod10/2, dotprod11/2, dotprod12/2, dotprod13/2, dotprod14/2, dotprod15/2, dotprod16/2, dotprod17/2, dotprod18/2, dotprod19/2, dotprod20/2, dotprod21/2, dotprod22/2, dotprod23/2, dotprod24/2, dotprod25/2, dotprod26/2, dotprod27/2, dotprod28/2, dotprod29/2, dotprod30/2
  dotprod1/1 -> Mux/1
  "IW{1,1}(2,:)'"/1 -> dotprod2/1
  dotprod2/1 -> Mux/2
  "IW{1,1}(3,:)'"/1 -> dotprod3/1
  dotprod3/1 -> Mux/3
  "IW{1,1}(4,:)'"/1 -> dotprod4/1
  dotprod4/1 -> Mux/4
  "IW{1,1}(5,:)'"/1 -> dotprod5/1
  dotprod5/1 -> Mux/5
  "IW{1,1}(6,:)'"/1 -> dotprod6/1
  dotprod6/1 -> Mux/6
  "IW{1,1}(7,:)'"/1 -> dotprod7/1
  dotprod7/1 -> Mux/7
  "IW{1,1}(8,:)'"/1 -> dotprod8/1
  dotprod8/1 -> Mux/8
  "IW{1,1}(9,:)'"/1 -> dotprod9/1
  dotprod9/1 -> Mux/9
  "IW{1,1}(10,:)'"/1 -> dotprod10/1
  dotprod10/1 -> Mux/10
  "IW{1,1}(11,:)'"/1 -> dotprod11/1
  dotprod11/1 -> Mux/11
  "IW{1,1}(12,:)'"/1 -> dotprod12/1
  dotprod12/1 -> Mux/12
  "IW{1,1}(13,:)'"/1 -> dotprod13/1
  dotprod13/1 -> Mux/13
  "IW{1,1}(14,:)'"/1 -> dotprod14/1
  dotprod14/1 -> Mux/14
  "IW{1,1}(15,:)'"/1 -> dotprod15/1
  dotprod15/1 -> Mux/15
  "IW{1,1}(16,:)'"/1 -> dotprod16/1
  dotprod16/1 -> Mux/16
  "IW{1,1}(17,:)'"/1 -> dotprod17/1
  dotprod17/1 -> Mux/17
  "IW{1,1}(18,:)'"/1 -> dotprod18/1
  dotprod18/1 -> Mux/18
  "IW{1,1}(19,:)'"/1 -> dotprod19/1
  dotprod19/1 -> Mux/19
  "IW{1,1}(20,:)'"/1 -> dotprod20/1
  dotprod20/1 -> Mux/20
  "IW{1,1}(21,:)'"/1 -> dotprod21/1
  dotprod21/1 -> Mux/21
  "IW{1,1}(22,:)'"/1 -> dotprod22/1
  dotprod22/1 -> Mux/22
  "IW{1,1}(23,:)'"/1 -> dotprod23/1
  dotprod23/1 -> Mux/23
  "IW{1,1}(24,:)'"/1 -> dotprod24/1
  dotprod24/1 -> Mux/24
  "IW{1,1}(25,:)'"/1 -> dotprod25/1
  dotprod25/1 -> Mux/25
  "IW{1,1}(26,:)'"/1 -> dotprod26/1
  dotprod26/1 -> Mux/26
  "IW{1,1}(27,:)'"/1 -> dotprod27/1
  dotprod27/1 -> Mux/27
  "IW{1,1}(28,:)'"/1 -> dotprod28/1
  dotprod28/1 -> Mux/28
  "IW{1,1}(29,:)'"/1 -> dotprod29/1
  dotprod29/1 -> Mux/29
  "IW{1,1}(30,:)'"/1 -> dotprod30/1
  dotprod30/1 -> Mux/30
  Mux/1 -> "iz{1,1}"/1

== system mrefrobotarm_modified_previous_y_previous_u_previous_ref_pert_2/m=0 sd=0.01/Layer 2/Delays 1 ==
  "p{2}" : Inport  PortDimensions=30
      mask Display: e = 0.06;c1 = [120 230 180]/255;c2 = ([120 230 180]+0)/(256+128);c3 = ([120 230 180]+128)/(256+128);patch([0 1 1 0],[0 0 1 1],c1);patch([0 1 1 1-e 1-e 0+e],[0 0 1 1-e 0+e 0+e],c2);patch([0 0 1 1-e 0+e 0+e],[0 1 1 1-e 1-e 0+e],c3);plot([0 1 1 0 0],[0 0 1 1 0]);
  mux : Mux  Inputs=1
      mask Display: e = 0.06;c1 = [120 150 230]/255;c2 = ([120 150 230]+0)/383;c3 = ([120 150 230]+128)/383;patch([0 1 1 0],[0 0 1 1],c1);patch([0 1 1 1-e 1-e 0+e],[0 0 1 1-e 0+e 0+e],c2);patch([0 0 1 1-e 0+e 0+e],[0 1 1 1-e 1-e 0+e],c3);plot([0 1 1 0 0],[0 0 1 1 0]);disp('Mux')
  "pd{2,1}" : Outport
      mask Display: e = 0.06;c1 = [120 230 180]/255;c2 = ([120 230 180]+0)/(256+128);c3 = ([120 230 180]+128)/(256+128);patch([0 1 1 0],[0 0 1 1],c1);patch([0 1 1 1-e 1-e 0+e],[0 0 1 1-e 0+e 0+e],c2);patch([0 0 1 1-e 0+e 0+e],[0 1 1 1-e 1-e 0+e],c3);plot([0 1 1 0 0],[0 0 1 1 0]);
  wires:
  "p{2}"/1 -> mux/1
  mux/1 -> "pd{2,1}"/1
